simulink model "Problem2"  (R2020a)
settings: Solver=VariableStepAuto  StartTime=0.0  StopTime=10.0  RelTol=1e-3
settings Model: Creator=HP  LastModifiedBy=HP

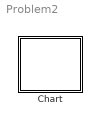
== system Problem2 ==
  Chart : Stateflow chart  TreatAsAtomicUnit=on

== stateflow chart Problem2/Chart ==
  state stop
    y1=Red;
    y2=Green;
  state stop_for_traffic
    y1=Red
    y2=Green;
  state stop_to_go
    y1=Red;
    y2=Green;
  state go_to_stop
    y1=Yellow;
    y2=Red;
  state o
    y1=Green;
    y2=Red;
  (default) -> stop
  stop -> stop_for_traffic : after(20,tick)
  stop_for_traffic -> stop_to_go : [sens]
  go_to_stop -> stop : after(3,tick)
  stop_to_go -> o : after(3,tick)
  o -> go_to_stop : after(10,tick)
